simulink model "2(A)"  (R2019b)
settings: Solver=VariableStepAuto  StartTime=0.0  StopTime=10.0  RelTol=1e-3
settings Model: Creator=tracy  LastModifiedBy=tracy

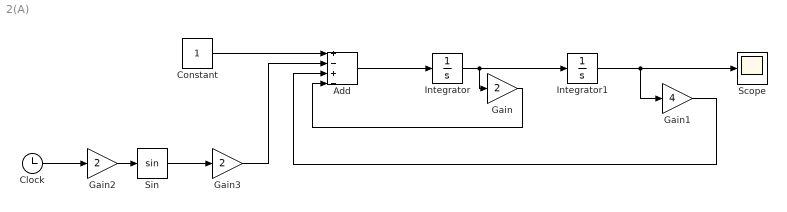
== system 2(A) ==
  Add : Sum  Inputs=+-+-
  Clock : Clock
  Constant : Constant
  Gain : Gain  Gain=2
  Gain1 : Gain  Gain=4
  Gain2 : Gain  Gain=2
  Gain3 : Gain  Gain=2
  Integrator : Integrator
  Integrator1 : Integrator
  Scope : Scope
  Sin : Trigonometry
  wires:
  Add/1 -> Integrator/1
  Integrator/1 -> Gain/1, Integrator1/1
  Gain/1 -> Add/4
  Integrator1/1 -> Gain1/1, Scope/1
  Gain1/1 -> Add/3
  Constant/1 -> Add/1
  Gain2/1 -> Sin/1
  Sin/1 -> Gain3/1
  Clock/1 -> Gain2/1
  Gain3/1 -> Add/2
